simulink model "DCmotor_Speed_Ctrl_SILS"  (R2021b)
settings: Solver=FixedStepAuto  StartTime=0.0  StopTime=20  FixedStep=Ts  RelTol=1e-3
values from neighbouring files (symbols this model uses):
  J = 0.02    [para.m]
  Kb = 0.1    [para.m]
  Kf = 0.01    [para.m]
  Ki = 50    [para.m]
  Km = 1    [para.m]
  Kp = 100    [para.m]
  L = 0.5    [para.m]
  R = 2    [para.m]
  Vlim = 12    [para.m]
  Wref = 100    [para.m]
settings Model: Creator=user  LastModifiedBy=user

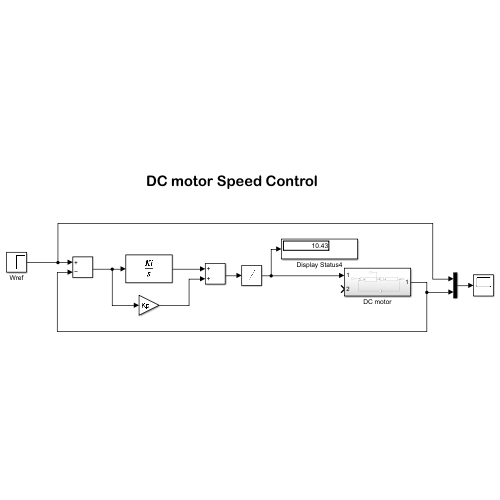
[thumbnail: Simulink's stored preview of the top-level diagram]
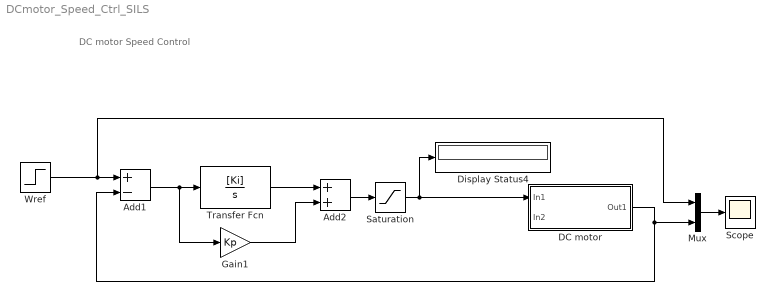
== system DCmotor_Speed_Ctrl_SILS ==
  note: DC motor Speed Control
  Add1 : Sum  Inputs=+-
  Add2 : Sum
  DC motor : Subsystem
  Display Status4 : Display
  Gain1 : Gain  Gain=Kp
  Mux : Mux  Inputs=2
  Saturation : Saturate  UpperLimit=Vlim  LowerLimit=0
  Scope : Scope
  Transfer Fcn : TransferFcn  Numerator=[Ki]  Denominator=[1 0]
  Wref : Step  Time=0  After=Wref  SampleTime=0
  wires:
  DC motor/1(Out1) -> Add1/2, Mux/2
  Transfer Fcn/1 -> Add2/1
  Gain1/1 -> Add2/2
  Wref/1 -> Mux/1, Add1/1
  Add1/1 -> Gain1/1, Transfer Fcn/1
  Add2/1 -> Saturation/1
  Mux/1 -> Scope/1
  Saturation/1 -> DC motor/1(In1), Display Status4/1

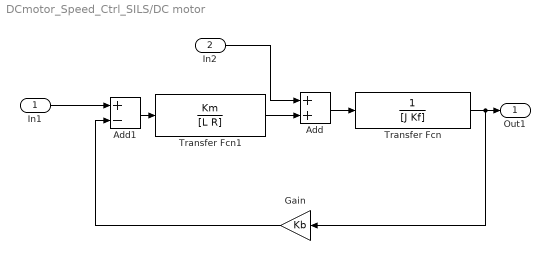
== system DCmotor_Speed_Ctrl_SILS/DC motor ==
  In1 : Inport
  In2 : Inport  Port=2
  Add : Sum
  Add1 : Sum  Inputs=+-
  Gain : Gain  Gain=Kb
  Transfer Fcn : TransferFcn  Denominator=[J Kf]
  Transfer Fcn1 : TransferFcn  Numerator=Km  Denominator=[L R]
  Out1 : Outport
  wires:
  Transfer Fcn1/1 -> Add/2
  Add/1 -> Transfer Fcn/1
  In2/1 -> Add/1
  Add1/1 -> Transfer Fcn1/1
  In1/1 -> Add1/1
  Transfer Fcn/1 -> Gain/1, Out1/1
  Gain/1 -> Add1/2
